simulink model "untitled"  (R2019b)
settings: Solver=VariableStepAuto  StartTime=0.0  StopTime=300  FixedStep=0.01  RelTol=1e-3
undefined symbols (not defined in the file): alpha1, alpha2, beta1, beta2, CaCO2_IC, CaO2_IC, Cbp, Cbv, Cep, Cev, Chp, Chv, Cla, Cmp, Cmv, Cpa, Cpp, Cps, Cpv, Cra, Csa, CsatCO2, CsatO2, Csp, Csv, CvCO2_IC, CvO2_IC, D1, D2, Dc, Dp, dt, Emaxlv, Emaxrv, f, fac_max, fac_min, facn, FICO2, FIO2, GcA, Gcf, GpA, Gpf, h1, h2, HR, K1, K1_tv, K2, K2_tv, kac, kElv, kErv, KH, KR, kRlv, kRrv, ksys, Kxp ... (+70)
libraries: fl_lib x42, nesl_utility x9, powerlib_meascontrol x1
(part 1 of 2)
settings Model: Creator=muratcangncr  LastModifiedBy=muratcangncr

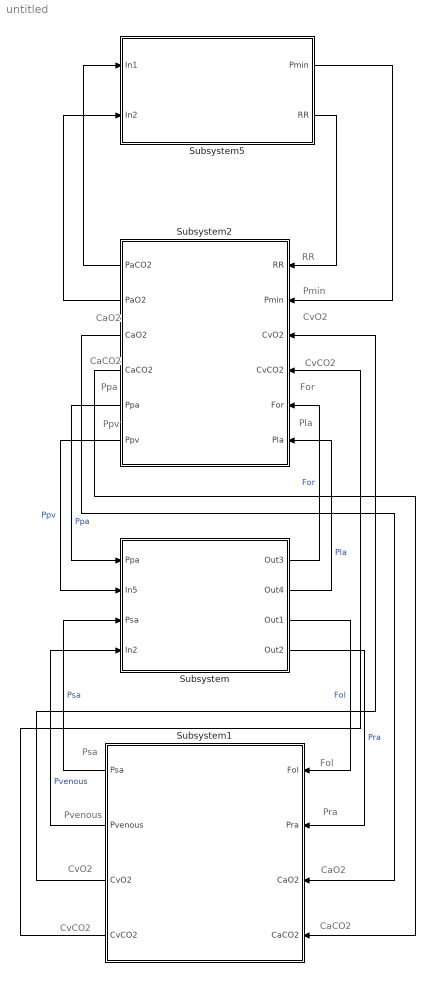
== system untitled ==
  note: Pmin
  note: RR
  note: Pvenous
  note: Psa
  note: Fol
  note: Pra
  note: CaO2
  note: CaCO2
  note: Ppa
  note: Ppv
  note: CvO2
  note: CvCO2
  note: For
  note: Pla
  note: CaO2
  note: CaCO2
  note: CvO2
  note: CvCO2
  Subsystem : Subsystem
      mask Display: image('C:\Users\muratcangncr\Desktop\MIT-Biorobotic-Heart-A1.jpg'); % Use "Edit Image" on toolstrip to change.
  Subsystem1 : Subsystem
      mask Display: image('C:\Users\muratcangncr\Desktop\systemic.jpg'); % Use "Edit Image" on toolstrip to change.
  Subsystem2 : Subsystem
      mask Display: image('C:\Users\muratcangncr\Desktop\pulmo.png'); % Use "Edit Image" on toolstrip to change.
  Subsystem5 : Subsystem
  wires:
  Subsystem/3(Out1) -> Subsystem1/1(Fol)  "Fol"
  Subsystem/4(Out2) -> Subsystem1/2(Pra)  "Pra"
  Subsystem1/1(Psa) -> Subsystem/3(Psa)  "Psa"
  Subsystem1/2(Pvenous) -> Subsystem/4(In2)  "Pvenous"
  Subsystem1/3(CvO2) -> Subsystem2/3(CvO2)
  Subsystem1/4(CvCO2) -> Subsystem2/4(CvCO2)
  Subsystem/1(Out3) -> Subsystem2/5(For)  "For"
  Subsystem/2(Out4) -> Subsystem2/6(Pla)  "Pla"
  Subsystem2/3(CaO2) -> Subsystem1/3(CaO2)
  Subsystem2/4(CaCO2) -> Subsystem1/4(CaCO2)
  Subsystem2/5(Ppa) -> Subsystem/1(Ppa)  "Ppa"
  Subsystem2/6(Ppv) -> Subsystem/2(In5)  "Ppv"
  Subsystem2/1(PaCO2) -> Subsystem5/1(In1)
  Subsystem2/2(PaO2) -> Subsystem5/2(In2)
  Subsystem5/1(Pmin) -> Subsystem2/2(Pmin)
  Subsystem5/2(RR) -> Subsystem2/1(RR)

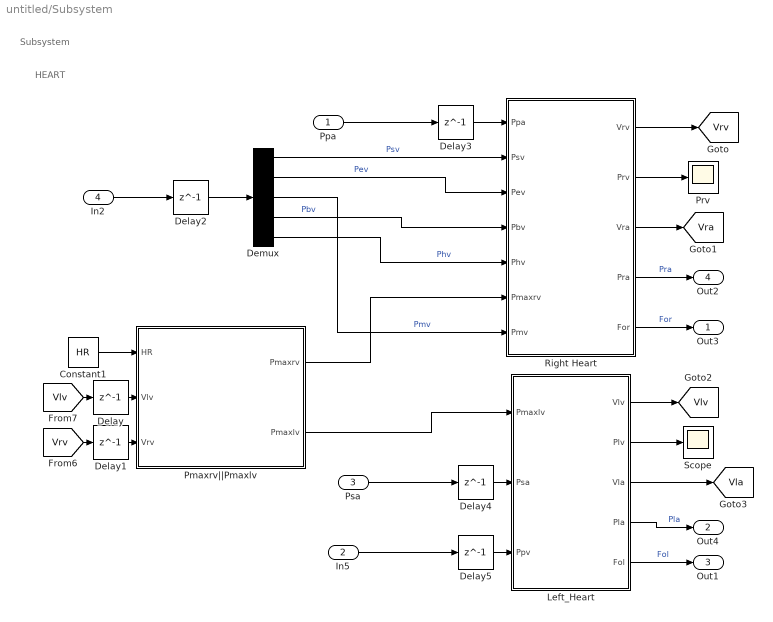
== system untitled/Subsystem ==
  note: Subsystem
  note: HEART
  Ppa : Inport
  In5 : Inport  Port=2
  Psa : Inport  Port=3
  In2 : Inport  Port=4
  Constant1 : Constant  Value=HR
  Delay{,1..5} (6 alike) : Delay  DelayLength=1  SampleTime=Tsamp
  Demux : Demux  Outputs=5
  "Left_Heart " : MATLAB Function  TreatAsAtomicUnit=on  SystemSampleTime=Tsamp
  Pmaxrv||Pmaxlv : MATLAB Function  TreatAsAtomicUnit=on  SystemSampleTime=Tsamp
  Prv : Scope
  Right Heart : MATLAB Function  TreatAsAtomicUnit=on  SystemSampleTime=Tsamp
  Scope : Scope
  Out3 : Outport
  Out4 : Outport  Port=2
  Out1 : Outport  Port=3
  Out2 : Outport  Port=4
  tag scope: Vla=global, Vlv=global, Vra=global, Vrv=global
  wires:
  Right Heart/3(Vra) -> [Vra]
  "Left_Heart "/3(Vla) -> [Vla]
  "Left_Heart "/2(Plv) -> Scope/1
  Demux/1 -> Right Heart/2(Psv)  "Psv"
  Demux/2 -> Right Heart/3(Pev)  "Pev"
  "Left_Heart "/1(Vlv) -> [Vlv]
  Right Heart/2(Prv) -> Prv/1
  Delay4/1 -> "Left_Heart "/2(Psa)
  Pmaxrv||Pmaxlv/2(Pmaxlv) -> "Left_Heart "/1(Pmaxlv)
  Constant1/1 -> Pmaxrv||Pmaxlv/1(HR)
  Pmaxrv||Pmaxlv/1(Pmaxrv) -> Right Heart/6(Pmaxrv)
  [Vlv] -> Delay/1
  Right Heart/5(For) -> Out3/1  "For"
  Right Heart/1(Vrv) -> [Vrv]
  Delay1/1 -> Pmaxrv||Pmaxlv/3(Vrv)
  Demux/5 -> Right Heart/5(Phv)  "Phv"
  [Vrv] -> Delay1/1
  Demux/3 -> Right Heart/7(Pmv)  "Pmv"
  Delay/1 -> Pmaxrv||Pmaxlv/2(Vlv)
  Demux/4 -> Right Heart/4(Pbv)  "Pbv"
  Delay5/1 -> "Left_Heart "/3(Ppv)
  Delay3/1 -> Right Heart/1(Ppa)
  Delay2/1 -> Demux/1
  In5/1 -> Delay5/1
  "Left_Heart "/4(Pla) -> Out4/1  "Pla"
  In2/1 -> Delay2/1
  Right Heart/4(Pra) -> Out2/1  "Pra"
  "Left_Heart "/5(Fol) -> Out1/1  "Fol"
  Ppa/1 -> Delay3/1
  Psa/1 -> Delay4/1

== system untitled/Subsystem1 ==
  Fol : Inport
  Pra : Inport  Port=2
  CaO2 : Inport  Port=3
  CaCO2 : Inport  Port=4
  Constant : Constant  Value=Vt0  VectorParams1D=off  SampleTime=Tsamp
  Display : Display
  Mean : powerlib_meascontrol/Measurements/Mean  Freq=1.2  Vinit=0  Ts=0
      settings: SourceProductName=Simscape Electrical
  Mux : Mux  Inputs=5
  Systemic Circ. : MATLAB Function  TreatAsAtomicUnit=on  SystemSampleTime=Tsamp
  Tissue Gas Exchange1 : Subsystem
  Psa : Outport
  Pvenous : Outport  Port=2
  CvO2 : Outport  Port=3
  CvCO2 : Outport  Port=4
  wires:
  Systemic Circ./6(Pbv) -> Mux/4
  [Vrv] -> Systemic Circ./3(Vrv)
  [Vpp] -> Systemic Circ./5(Vpp)
  Systemic Circ./5(Pmv) -> Mux/3
  [Vlv] -> Systemic Circ./8(Vlv)
  [Vla] -> Systemic Circ./10(Vla)
  Systemic Circ./4(Pev) -> Mux/2
  Systemic Circ./7(Phv) -> Mux/5
  [Vpv] -> Systemic Circ./7(Vpv)
  Systemic Circ./3(Psv) -> Mux/1  "Psv"
  [Vps] -> Systemic Circ./6(Vps)
  [Vpa] -> Systemic Circ./4(Vpa)
  Fol/1 -> Systemic Circ./1(Fol)
  Systemic Circ./1(Fsa) -> Tissue Gas Exchange1/3(Fs), Mean/1
  Constant/1 -> Systemic Circ./9(Vtotal)
  Mean/1 -> Display/1
  Pra/1 -> Systemic Circ./2(Pra)
  Tissue Gas Exchange1/2(CvCO2) -> CvCO2/1  "CvCO2"
  [Vra] -> Systemic Circ./11(Vra)
  CaCO2/1 -> Tissue Gas Exchange1/1(CaCO2)  "CaCO2"
  Systemic Circ./2(Psa) -> Psa/1  "Psa"
  Mux/1 -> Pvenous/1  "Pvenous"
  CaO2/1 -> Tissue Gas Exchange1/2(CaO2)  "CaO2"
  Tissue Gas Exchange1/1(CvO2) -> CvO2/1  "CvO2"

== system untitled/Subsystem2 ==
  RR : Inport
  Pmin : Inport  Port=2
  CvO2 : Inport  Port=3
  CvCO2 : Inport  Port=4
  For : Inport  Port=5
  Pla : Inport  Port=6
  Pulmonary : MATLAB Function  TreatAsAtomicUnit=on  SystemSampleTime=Tsamp
  Scope : Scope
  The lungs : Subsystem
  PaCO2 : Outport
  PaO2 : Outport  Port=2
  CaO2 : Outport  Port=3
  CaCO2 : Outport  Port=4
  Ppa : Outport  Port=5
  Ppv : Outport  Port=6
  tag scope: Vpa=global, Vpp=global, Vps=global, Vpv=global
  wires:
  Pulmonary/4(Vpv) -> [Vpv]
  Pulmonary/9(Fps) -> The lungs/2(Fps)
  For/1 -> Pulmonary/1(For)
  Pmin/1 -> The lungs/6(Pmin)
  CvCO2/1 -> The lungs/4(CvCO2)
  Pulmonary/5(Ppa) -> Ppa/1  "Ppa"
  Pla/1 -> Pulmonary/2(Pla)
  Pulmonary/3(Vps) -> [Vps]
  Pulmonary/1(Vpa) -> [Vpa]
  Pulmonary/2(Vpp) -> [Vpp]
  The lungs/2(PaCO2) -> PaCO2/1
  Pulmonary/7(Fpa) -> Scope/1
  Pulmonary/8(Fpp) -> The lungs/1(Fpp)
  RR/1 -> The lungs/5(RR)
  The lungs/1(PaO2) -> PaO2/1
  Pulmonary/6(Ppv) -> Ppv/1  "Ppv"
  The lungs/3(CaCO2) -> CaCO2/1
  The lungs/4(CaO2) -> CaO2/1
  CvO2/1 -> The lungs/3(CvO2)

== system untitled/Subsystem5 ==
  In1 : Inport
  In2 : Inport  Port=2
  Add1 : Sum  Inputs=+++
  Add5 : Sum  Inputs=+--
  Constant : Constant  Value=Pmin0
  Constant1 : Constant  Value=RR0
  MATLAB Function : MATLAB Function  TreatAsAtomicUnit=on
  Subsystem3 : Subsystem
  Subsystem4 : Subsystem
  Pmin : Outport
  RR : Outport  Port=2
  wires:
  Subsystem3/1(dRRp) -> Add1/3
  Add1/1 -> RR/1
  In1/1 -> Subsystem4/1(In1), MATLAB Function/1(PaCO2)
  In2/1 -> MATLAB Function/2(PaO2)
  MATLAB Function/1(fac) -> Subsystem3/1(In1)
  Subsystem4/1(dRRc) -> Add1/2
  Add5/1 -> Pmin/1
  Constant1/1 -> Add1/1
  Subsystem3/2(dPminP) -> Add5/3
  Subsystem4/2(dPminc) -> Add5/2
  Constant/1 -> Add5/1

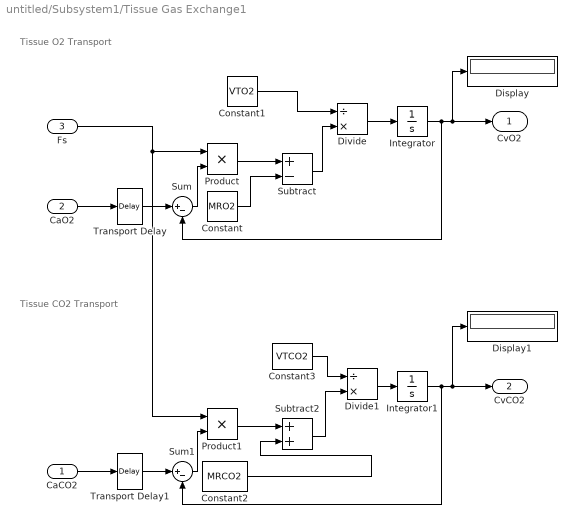
== system untitled/Subsystem1/Tissue Gas Exchange1 ==
  note: Tissue O2 Transport
  note: Tissue CO2 Transport
  CaCO2 : Inport
  CaO2 : Inport  Port=2
  Fs : Inport  Port=3
  Constant : Constant  Value=MRO2
  Constant1 : Constant  Value=VTO2
  Constant2 : Constant  Value=MRCO2
  Constant3 : Constant  Value=VTCO2
  Display : Display
  Display1 : Display
  Divide : Product  Inputs=/*
  Divide1 : Product  Inputs=/*
  Integrator : Integrator  InitialCondition=CvO2_IC
  Integrator1 : Integrator  InitialCondition=CvCO2_IC
  Product : Product
  Product1 : Product
  Subtract : Sum  Inputs=+-
  Subtract2 : Sum
  Sum : Sum  Inputs=|+-
  Sum1 : Sum  Inputs=|+-
  Transport Delay : TransportDelay  DelayTime=Tau_LT  InitialOutput=CaO2_IC
  Transport Delay1 : TransportDelay  DelayTime=Tau_LT  InitialOutput=CaCO2_IC
  CvO2 : Outport  VectorParamsAs1DForOutWhenUnconnected=off
  CvCO2 : Outport  Port=2  VectorParamsAs1DForOutWhenUnconnected=off
  wires:
  CaO2/1 -> Transport Delay/1
  Transport Delay/1 -> Sum/1
  Sum/1 -> Product/2
  Product/1 -> Subtract/1
  Divide/1 -> Integrator/1
  Integrator/1 -> Sum/2, Display/1, CvO2/1
  Subtract/1 -> Divide/2
  Constant1/1 -> Divide/1
  Product1/1 -> Subtract2/1
  Transport Delay1/1 -> Sum1/1
  Sum1/1 -> Product1/2
  Fs/1 -> Product1/1, Product/1
  Constant3/1 -> Divide1/1
  Integrator1/1 -> Sum1/2, CvCO2/1, Display1/1
  Subtract2/1 -> Divide1/2
  Divide1/1 -> Integrator1/1
  CaCO2/1 -> Transport Delay1/1
  Constant/1 -> Subtract/2
  Constant2/1 -> Subtract2/2

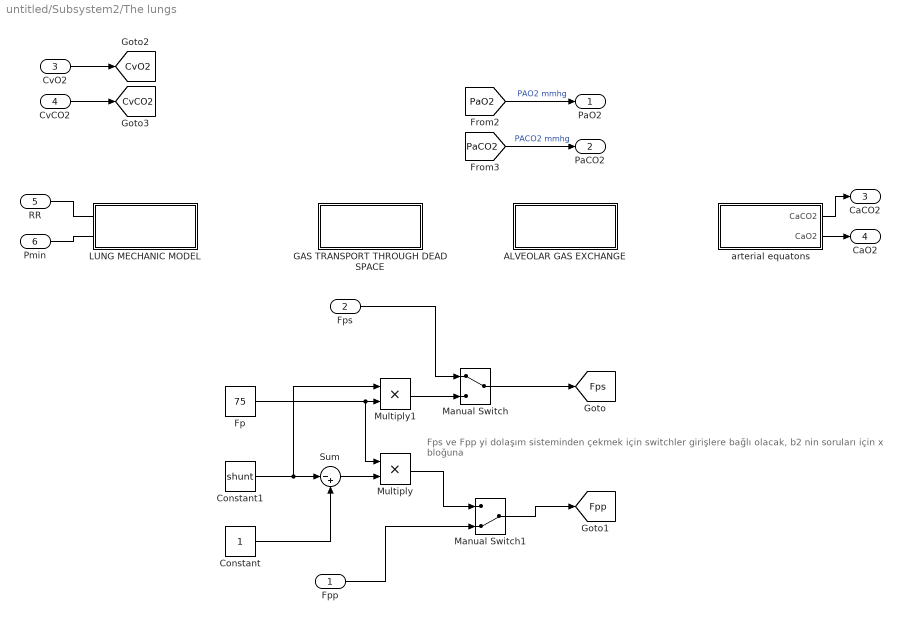
== system untitled/Subsystem2/The lungs ==
  note: Fps ve Fpp yi dolaşım sisteminden çekmek için switchler girişlere bağlı olacak, b2 nin soruları için x bloğuna
  Fpp : Inport
  Fps : Inport  Port=2
  CvO2 : Inport  Port=3
  CvCO2 : Inport  Port=4
  RR : Inport  Port=5
  Pmin : Inport  Port=6
  ALVEOLAR GAS EXCHANGE : Subsystem
  Constant : Constant
  Constant1 : Constant  Value=shunt
  Fp : Constant  Value=75
  GAS TRANSPORT THROUGH DEAD SPACE : Subsystem
  LUNG MECHANIC MODEL : Subsystem
  Manual Switch : ManualSwitch
  Manual Switch1 : ManualSwitch  CurrentSetting=0
  Multiply : Product
  Multiply1 : Product
  Sum : Sum  Inputs=|-+
  arterial equatons : Subsystem
  PaO2 : Outport  VectorParamsAs1DForOutWhenUnconnected=off
  PaCO2 : Outport  Port=2  VectorParamsAs1DForOutWhenUnconnected=off
  CaCO2 : Outport  Port=3
  CaO2 : Outport  Port=4
  tag scope: CvCO2=global, CvO2=global, Fpp=global, Fps=global
  wires:
  Pmin/1 -> ?
  RR/1 -> ?
  CvO2/1 -> [CvO2]
  CvCO2/1 -> [CvCO2]
  Constant/1 -> Sum/2
  Fpp/1 -> Manual Switch1/2
  Constant1/1 -> Multiply1/1, Sum/1
  Sum/1 -> Multiply/2
  Fp/1 -> Multiply/1, Multiply1/2
  Manual Switch1/1 -> [Fpp]
  Multiply1/1 -> Manual Switch/2
  Manual Switch/1 -> [Fps]
  Fps/1 -> Manual Switch/1
  Multiply/1 -> Manual Switch1/1
  [PaCO2] -> PaCO2/1  "PACO2 mmhg"
  [PaO2] -> PaO2/1  "PAO2 mmhg"
  arterial equatons/1(CaCO2) -> CaCO2/1
  arterial equatons/2(CaO2) -> CaO2/1

== system untitled/Subsystem5/Subsystem3 ==
  In1 : Inport
  Add2 : Sum  Inputs=+-
  Add3 : Sum  Inputs=+-
  Add4 : Sum  Inputs=+-
  Constant5 : Constant  Value=facn
  Constant6 : Constant  Value=GpA
  Constant7 : Constant  Value=TaupA
  Constant8 : Constant  Value=Gpf
  Constant9 : Constant  Value=Taupf
  Divide2 : Product  Inputs=*/
  Divide3 : Product  Inputs=*/
  Integrator2 : Integrator
  Integrator3 : Integrator
  Product2 : Product
  Product4 : Product
  Transport Delay1 : TransportDelay  DelayTime=Dp
  dRRp : Outport
  dPminP : Outport  Port=2
  wires:
  Add4/1 -> Divide3/1
  Constant7/1 -> Divide2/2
  Constant9/1 -> Divide3/2
  Product4/1 -> Add4/1
  Product2/1 -> Add3/1
  Integrator3/1 -> dRRp/1, Add4/2  "dRRp"
  Integrator2/1 -> dPminP/1, Add3/2  "dPminP"
  Add2/1 -> Product4/2, Product2/1
  Transport Delay1/1 -> Add2/1
  Constant8/1 -> Product4/1
  Divide2/1 -> Integrator2/1
  Add3/1 -> Divide2/1
  Divide3/1 -> Integrator3/1
  In1/1 -> Transport Delay1/1
  Constant5/1 -> Add2/2
  Constant6/1 -> Product2/2

== system untitled/Subsystem5/Subsystem4 ==
  In1 : Inport
  Add1 : Sum  Inputs=+-
  Add5 : Sum  Inputs=+-
  Constant : Constant  Value=PaCO2n
  Constant1 : Constant  Value=GcA
  Constant2 : Constant  Value=TaucA
  Constant3 : Constant  Value=Gcf
  Constant4 : Constant  Value=Taucf
  Divide : Product  Inputs=*/
  Divide1 : Product  Inputs=*/
  Integrator : Integrator
  Integrator1 : Integrator
  Product1 : Product
  Product3 : Product
  Sum : Sum  Inputs=-+|
  Transport Delay : TransportDelay  DelayTime=Dc
  dRRc : Outport
  dPminc : Outport  Port=2
  wires:
  Divide/1 -> Integrator/1
  Constant3/1 -> Product1/2
  Integrator1/1 -> dRRc/1, Add1/2  "dRRc"
  Add5/1 -> Divide/1
  Add1/1 -> Divide1/1
  Integrator/1 -> dPminc/1, Add5/2  "dPminc"
  Sum/1 -> Product1/1, Product3/1  "Uc"
  Constant1/1 -> Product3/2
  Product3/1 -> Add5/1
  Constant/1 -> Sum/1
  Constant2/1 -> Divide/2
  Divide1/1 -> Integrator1/1
  Constant4/1 -> Divide1/2
  Product1/1 -> Add1/1
  Transport Delay/1 -> Sum/2
  In1/1 -> Transport Delay/1

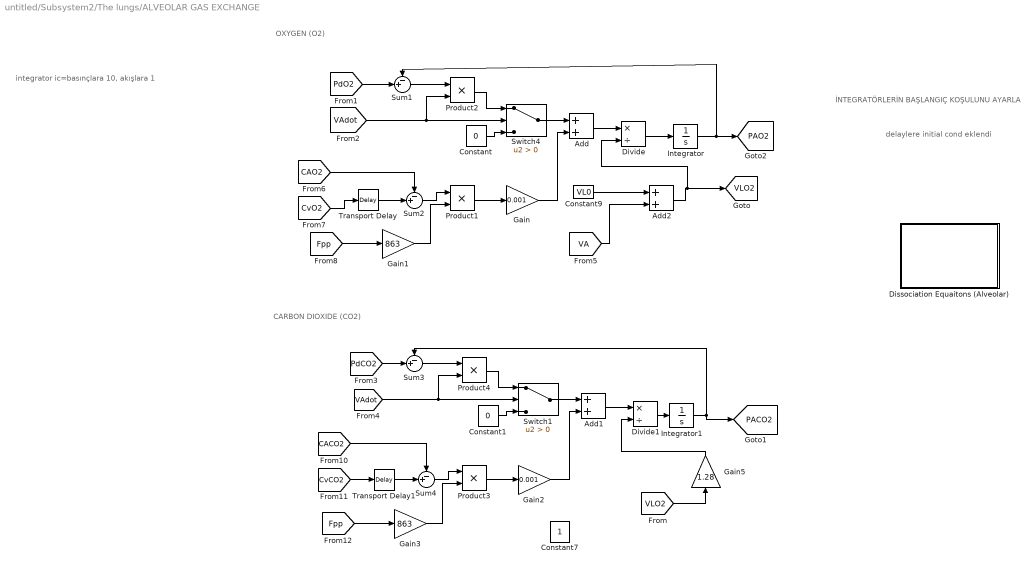
== system untitled/Subsystem2/The lungs/ALVEOLAR GAS EXCHANGE ==
  note: integrator ic=basınçlara 10, akışlara 1
  note: delaylere initial cond eklendi
  note: İNTEGRATÖRLERİN BAŞLANGIÇ KOŞULUNU AYARLA
  note: CARBON DIOXIDE (CO2)
  note: OXYGEN (O2)
  Add : Sum
  Add1 : Sum
  Add2 : Sum
  Constant : Constant  Value=0
  Constant1 : Constant  Value=0
  Constant7 : Constant
  Constant9 : Constant  Value=VL0
  Dissociation Equaitons (Alveolar) : Subsystem
  Divide : Product  Inputs=*/
  Divide1 : Product  Inputs=*/
  Gain : Gain  Gain=0.001
  Gain1 : Gain  Gain=863
  Gain2 : Gain  Gain=0.001
  Gain3 : Gain  Gain=863
  Gain5 : Gain  Gain=1.28
  Integrator : Integrator  InitialCondition=10
  Integrator1 : Integrator  InitialCondition=10
  Product{1..4} (4 alike) : Product
  Sum{1..4} (4 alike) : Sum  Inputs=-+|
  Switch1 : Switch  Criteria=u2 > Threshold
  Switch4 : Switch  Criteria=u2 > Threshold
  Transport Delay : TransportDelay  DelayTime=Tau_TL  InitialOutput=CvO2_IC
  Transport Delay1 : TransportDelay  DelayTime=Tau_TL  InitialOutput=CvCO2_IC
  tag scope: PACO2=global, PAO2=global, VLO2=global
  wires:
  [VAdot] -> Switch4/2, Product2/2
  Divide/1 -> Integrator/1
  [PdO2] -> Sum1/2
  Sum1/1 -> Product2/1
  Product2/1 -> Switch4/1
  Integrator/1 -> [PAO2], Sum1/1
  Constant/1 -> Switch4/3
  Switch4/1 -> Add/1
  Add/1 -> Divide/1
  Product1/1 -> Gain/1
  Gain/1 -> Add/2
  Sum2/1 -> Product1/1
  Gain1/1 -> Product1/2
  [CAO2] -> Sum2/1
  [CvO2] -> Transport Delay/1
  [Fpp] -> Gain1/1
  Transport Delay/1 -> Sum2/2
  Divide1/1 -> Integrator1/1
  Constant1/1 -> Switch1/3
  [VAdot] -> Switch1/2, Product4/2
  Product3/1 -> Gain2/1
  Sum3/1 -> Product4/1
  [PdCO2] -> Sum3/2
  Product4/1 -> Switch1/1
  Integrator1/1 -> [PACO2], Sum3/1
  Transport Delay1/1 -> Sum4/2
  [CACO2] -> Sum4/1
  Switch1/1 -> Add1/1
  Sum4/1 -> Product3/1
  [Fpp] -> Gain3/1
  [CvCO2] -> Transport Delay1/1
  Gain2/1 -> Add1/2
  Gain3/1 -> Product3/2
  Add1/1 -> Divide1/1
  [VA] -> Add2/2
  Constant9/1 -> Add2/1
  Add2/1 -> Divide/2, [VLO2]
  Gain5/1 -> Divide1/2
  [VLO2] -> Gain5/1

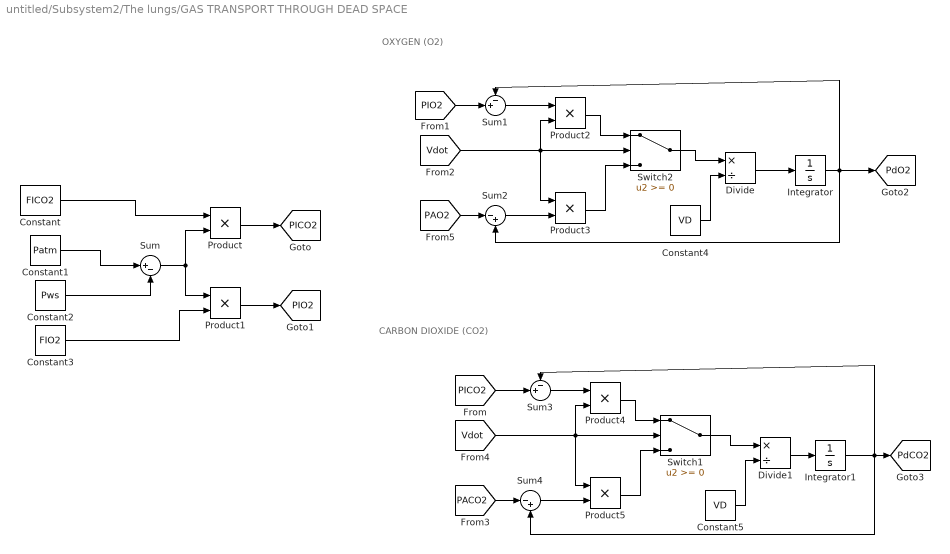
== system untitled/Subsystem2/The lungs/GAS TRANSPORT THROUGH DEAD SPACE ==
  note: CARBON DIOXIDE (CO2)
  note: OXYGEN (O2)
  Constant : Constant  Value=FICO2
  Constant1 : Constant  Value=Patm
  Constant2 : Constant  Value=Pws
  Constant3 : Constant  Value=FIO2
  Constant4 : Constant  Value=VD
  Constant5 : Constant  Value=VD
  Divide : Product  Inputs=*/
  Divide1 : Product  Inputs=*/
  Integrator : Integrator  InitialCondition=PdO2_IC
  Integrator1 : Integrator  InitialCondition=PdCO2_IC
  Product{,1..5} (6 alike) : Product
  Sum : Sum  Inputs=|+-
  Sum1 : Sum  Inputs=-+|
  Sum2 : Sum  Inputs=|-+
  Sum3 : Sum  Inputs=-+|
  Sum4 : Sum  Inputs=|-+
  Switch1 : Switch
  Switch2 : Switch
  tag scope: PICO2=global, PIO2=global, PdCO2=global, PdO2=global
  wires:
  Constant1/1 -> Sum/1
  Constant2/1 -> Sum/2
  Constant/1 -> Product/1
  Constant3/1 -> Product1/2
  Sum/1 -> Product1/1, Product/2
  Product/1 -> [PICO2]
  Product1/1 -> [PIO2]
  [PIO2] -> Sum1/2
  Sum1/1 -> Product2/1
  Product2/1 -> Switch2/1
  Switch2/1 -> Divide/1
  Constant4/1 -> Divide/2
  Divide/1 -> Integrator/1
  Integrator/1 -> Sum2/2, [PdO2], Sum1/1
  Sum2/1 -> Product3/2
  [Vdot] -> Switch2/2, Product3/1, Product2/2
  Product3/1 -> Switch2/3
  Product5/1 -> Switch1/3
  Divide1/1 -> Integrator1/1
  [PICO2] -> Sum3/2
  Switch1/1 -> Divide1/1
  Sum4/1 -> Product5/2
  [Vdot] -> Switch1/2, Product5/1, Product4/2
  Constant5/1 -> Divide1/2
  Sum3/1 -> Product4/1
  Product4/1 -> Switch1/1
  Integrator1/1 -> Sum4/2, [PdCO2], Sum3/1
  [PACO2] -> Sum4/1
  [PAO2] -> Sum2/1

== system untitled/Subsystem2/The lungs/LUNG MECHANIC MODEL ==
  Subsystem : Subsystem
  VAdot : Subsystem
  ab : Subsystem
  c : Subsystem
  d : Subsystem

== system untitled/Subsystem2/The lungs/arterial equatons ==
  CONSTANTRATION : Subsystem
  PARTİAL PRESSURES : Subsystem
  CaCO2 : Outport
  CaO2 : Outport  Port=2
  wires:
  CONSTANTRATION/1(CaCO2) -> CaCO2/1
  CONSTANTRATION/2(CaO2) -> CaO2/1

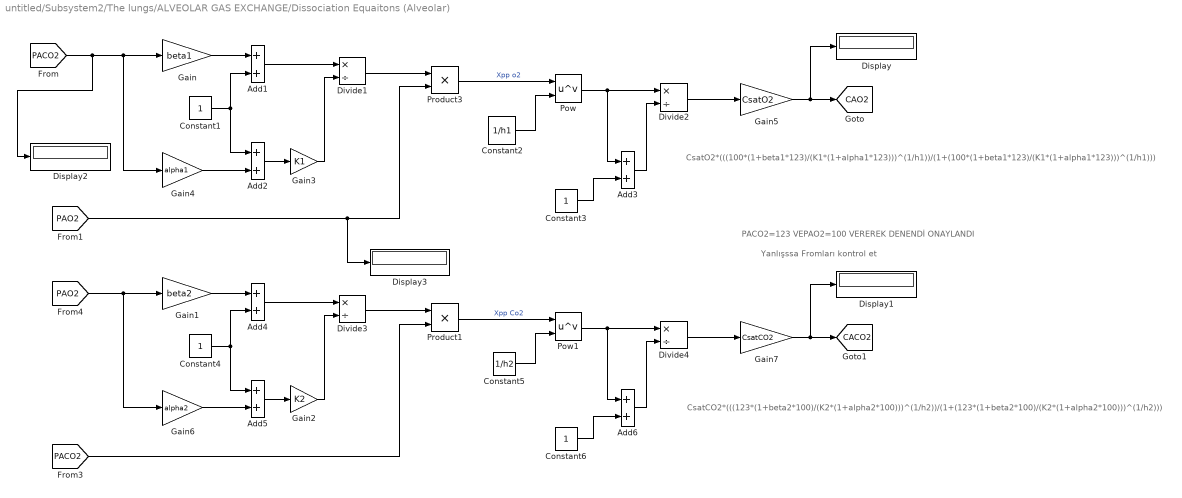
== system untitled/Subsystem2/The lungs/ALVEOLAR GAS EXCHANGE/Dissociation Equaitons (Alveolar) ==
  note: Yanlışssa Fromları kontrol et
  note: CsatO2*(((100*(1+beta1*123)/(K1*(1+alpha1*123)))^(1/h1))/(1+(100*(1+beta1*123)/(K1*(1+alpha1*123)))^(1/h1)))
  note: CsatCO2*(((123*(1+beta2*100)/(K2*(1+alpha2*100)))^(1/h2))/(1+(123*(1+beta2*100)/(K2*(1+alpha2*100)))^(1/h2)))
  note: PACO2=123 VEPAO2=100 VEREREK DENENDİ ONAYLANDI
  Add{1..6} (6 alike) : Sum
  Constant{1,3..4,6} (4 alike) : Constant
  Constant2 : Constant  Value=1/h1
  Constant5 : Constant  Value=1/h2
  Display{,1..3} (4 alike) : Display
  Divide{1..4} (4 alike) : Product  Inputs=*/
  Gain : Gain  Gain=beta1
  Gain1 : Gain  Gain=beta2
  Gain2 : Gain  Gain=K2
  Gain3 : Gain  Gain=K1
  Gain4 : Gain  Gain=alpha1
  Gain5 : Gain  Gain=CsatO2
  Gain6 : Gain  Gain=alpha2
  Gain7 : Gain  Gain=CsatCO2
  Pow : Math  Operator=pow  RndMeth=Zero  SaturateOnIntegerOverflow=on
  Pow1 : Math  Operator=pow  RndMeth=Zero  SaturateOnIntegerOverflow=on
  Product1 : Product
  Product3 : Product
  tag scope: CACO2=global, CAO2=global
  wires:
  [PACO2] -> Display2/1, Gain4/1, Gain/1
  Gain/1 -> Add1/1
  Constant1/1 -> Add2/1, Add1/2
  Add1/1 -> Divide1/1
  Gain3/1 -> Divide1/2
  Add2/1 -> Gain3/1
  Gain4/1 -> Add2/2
  Divide1/1 -> Product3/1
  [PAO2] -> Display3/1, Product3/2
  Product3/1 -> Pow/1  "Xpp o2"
  Constant2/1 -> Pow/2
  Pow/1 -> Add3/1, Divide2/1
  Constant3/1 -> Add3/2
  Add3/1 -> Divide2/2
  Divide2/1 -> Gain5/1
  Gain5/1 -> Display/1, [CAO2]
  Divide3/1 -> Product1/1
  [PACO2] -> Product1/2
  Add5/1 -> Gain2/1
  Gain6/1 -> Add5/2
  Constant4/1 -> Add5/1, Add4/2
  [PAO2] -> Gain6/1, Gain1/1
  Gain2/1 -> Divide3/2
  Gain1/1 -> Add4/1
  Pow1/1 -> Add6/1, Divide4/1
  Constant5/1 -> Pow1/2
  Gain7/1 -> Display1/1, [CACO2]
  Add6/1 -> Divide4/2
  Constant6/1 -> Add6/2
  Product1/1 -> Pow1/1  "Xpp Co2"
  Add4/1 -> Divide3/1
  Divide4/1 -> Gain7/1

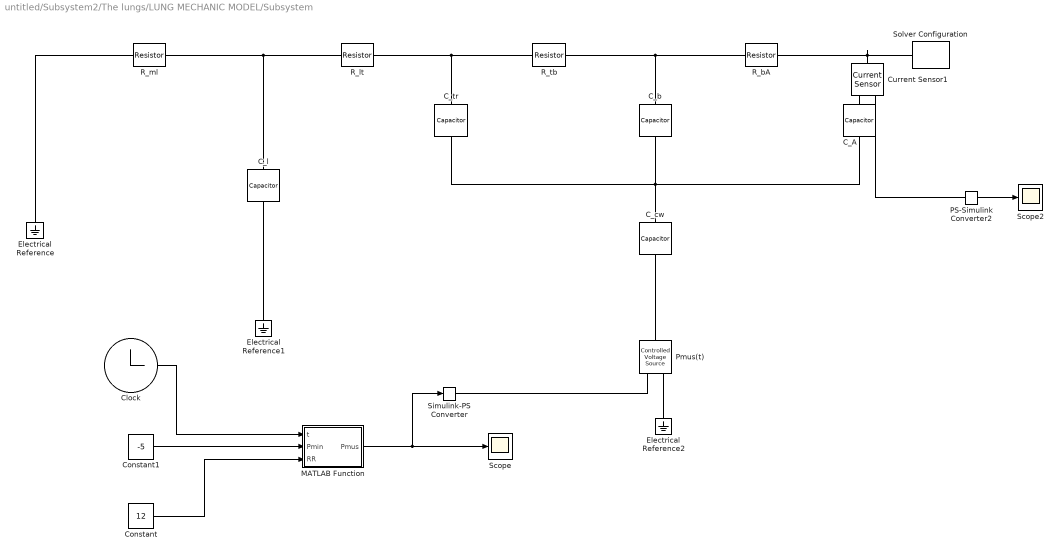
== system untitled/Subsystem2/The lungs/LUNG MECHANIC MODEL/Subsystem ==
  C_A : fl_lib/Electrical/Electrical Elements/Capacitor  c=0.175 F  r=0 Ohm  g=0 1/Ohm  i_specify=off  i_priority=None  i=0 A  i_nominal_specify=off  i_nominal_unit=A  i_nominal_value=1  v_specify=off  v_priority=None  v=0 V  v_nominal_specify=off  v_nominal_unit=V  v_nominal_value=1  vc_specify=off  vc_priority=High  vc=0 V  vc_nominal_specify=off  vc_nominal_unit=V  vc_nominal_value=1
  C_b : fl_lib/Electrical/Electrical Elements/Capacitor  c=0.0131 F  r=0 Ohm  g=0 1/Ohm  i_specify=off  i_priority=None  i=0 A  i_nominal_specify=off  i_nominal_unit=A  i_nominal_value=1  v_specify=off  v_priority=None  v=0 V  v_nominal_specify=off  v_nominal_unit=V  v_nominal_value=1  vc_specify=off  vc_priority=High  vc=0 V  vc_nominal_specify=off  vc_nominal_unit=V  vc_nominal_value=1
  C_cw : fl_lib/Electrical/Electrical Elements/Capacitor  c=0.2 F  r=0 Ohm  g=0 1/Ohm  i_specify=off  i_priority=None  i=0 A  i_nominal_specify=off  i_nominal_unit=A  i_nominal_value=1  v_specify=off  v_priority=None  v=0 V  v_nominal_specify=off  v_nominal_unit=V  v_nominal_value=1  vc_specify=off  vc_priority=High  vc=0 V  vc_nominal_specify=off  vc_nominal_unit=V  vc_nominal_value=1
  C_l : fl_lib/Electrical/Electrical Elements/Capacitor  c=0.00127 F  r=0 Ohm  g=0 1/Ohm  i_specify=off  i_priority=None  i=0 A  i_nominal_specify=off  i_nominal_unit=A  i_nominal_value=1  v_specify=off  v_priority=None  v=0 V  v_nominal_specify=off  v_nominal_unit=V  v_nominal_value=1  vc_specify=off  vc_priority=High  vc=0 V  vc_nominal_specify=off  vc_nominal_unit=V  vc_nominal_value=1
  C_tr : fl_lib/Electrical/Electrical Elements/Capacitor  c=0.00238 F  r=0 Ohm  g=0 1/Ohm  i_specify=off  i_priority=None  i=0 A  i_nominal_specify=off  i_nominal_unit=A  i_nominal_value=1  v_specify=off  v_priority=None  v=0 V  v_nominal_specify=off  v_nominal_unit=V  v_nominal_value=1  vc_specify=off  vc_priority=High  vc=0 V  vc_nominal_specify=off  vc_nominal_unit=V  vc_nominal_value=1
  Clock : Clock
      settings: Decimation=60
  Constant : Constant  Value=12
  Constant1 : Constant  Value=-5
  Current Sensor1 : fl_lib/Electrical/Electrical Sensors/Current Sensor
  Electrical Reference : fl_lib/Electrical/Electrical Elements/Electrical Reference
  Electrical Reference1 : fl_lib/Electrical/Electrical Elements/Electrical Reference
  Electrical Reference2 : fl_lib/Electrical/Electrical Elements/Electrical Reference
  MATLAB Function : MATLAB Function  TreatAsAtomicUnit=on
  PS-Simulink Converter2 : nesl_utility/PS-Simulink Converter  PhysicalDomain=network_engine_domain  SubClassName=ps_output  LeftPortType=input  RightPortType=output  PseudoPeriodic=off  Frequencies=[]  Unit=1  AffineConversion=off
  Pmus(t) : fl_lib/Electrical/Electrical Sources/Controlled Voltage Source
  R_bA : fl_lib/Electrical/Electrical Elements/Resistor  R=0.0817 Ohm  i_specify=off  i_priority=None  i=0 A  i_nominal_specify=off  i_nominal_unit=A  i_nominal_value=1  v_specify=off  v_priority=None  v=0 V  v_nominal_specify=off  v_nominal_unit=V  v_nominal_value=1
  R_lt : fl_lib/Electrical/Electrical Elements/Resistor  R=0.3369 Ohm  i_specify=off  i_priority=None  i=0 A  i_nominal_specify=off  i_nominal_unit=A  i_nominal_value=1  v_specify=off  v_priority=None  v=0 V  v_nominal_specify=off  v_nominal_unit=V  v_nominal_value=1
  R_ml : fl_lib/Electrical/Electrical Elements/Resistor  R=1.021 Ohm  i_specify=off  i_priority=None  i=0 A  i_nominal_specify=off  i_nominal_unit=A  i_nominal_value=1  v_specify=off  v_priority=None  v=0 V  v_nominal_specify=off  v_nominal_unit=V  v_nominal_value=1
  R_tb : fl_lib/Electrical/Electrical Elements/Resistor  R=0.3063 Ohm  i_specify=off  i_priority=None  i=0 A  i_nominal_specify=off  i_nominal_unit=A  i_nominal_value=1  v_specify=off  v_priority=None  v=0 V  v_nominal_specify=off  v_nominal_unit=V  v_nominal_value=1
  Scope : Scope
  Scope2 : Scope
  Simulink-PS Converter : nesl_utility/Simulink-PS Converter  PhysicalDomain=network_engine_domain  SubClassName=ps_input  LeftPortType=input  RightPortType=output  PseudoPeriodic=off  Frequencies=[]  NoiseDistribution=none  NoiseParameters=[]  Unit=1  AffineConversion=off  FilteringAndDerivatives=provide  SimscapeFilterOrder=1  InputFilterTimeConstant=0.001  UdotUserProvided=0
  Solver Configuration : nesl_utility/Solver Configuration  PhysicalDomain=network_engine_domain  SubClassName=solver  LeftPortType=input  RightPortType=generic  Tones=[]  Harmonics=[]  SimulateNoise=off  Profile=off  UseLocalSampling=off  EnableSwitchedLinearOptims=on  FrequencyDomain=off  UseCCode=off  RelTol=0.001  AbsTol=1e-06  MinStep=1e-09  ToWorkspace=off  RevertToSquareIcSolve=off  NumHomotopyIterations=100  PhasorMode=off  PhasorModeNumHarmonics=1  DoDC=off  ResidualTolerance=1e-09  UseLocalSolver=off  LocalSolverChoice=NE_BACKWARD_EULER_ADVANCER  LocalSolverSampleTime=0.001  DoFixedCost=off  MaxNonlinIter=3  MaxModeIter=2  LinearAlgebra=auto  EquationFormulation=NE_TIME_EF  DelaysMemoryBudget=1024  AutomaticFiltering=on  FilteringTimeConstant=0.001  PartitionStorageMethod=AS_NEEDED  PartitionMemoryBudget=1024  PartitionMethod=FAST
  wires:
  Constant/1 -> MATLAB Function/3(RR)
  MATLAB Function/1(Pmus) -> Scope/1, Simulink-PS Converter/1
  Constant1/1 -> MATLAB Function/2(Pmin)
  Clock/1 -> MATLAB Function/1(t)
  PS-Simulink Converter2/1 -> Scope2/1
  connections:
  R_lt/LConn1 -- R_ml/RConn1 -- C_l/LConn1
  C_A/RConn1 -- C_tr/RConn1 -- C_cw/LConn1 -- C_b/RConn1
  R_tb/LConn1 -- R_lt/RConn1 -- C_tr/LConn1
  Solver Configuration/RConn1 -- R_bA/RConn1 -- Current Sensor1/LConn1
  R_bA/LConn1 -- R_tb/RConn1 -- C_b/LConn1
  Current Sensor1/RConn1 -- PS-Simulink Converter2/LConn1
  R_ml/LConn1 -- Electrical Reference/LConn1
  Simulink-PS Converter/RConn1 -- Pmus(t)/RConn1
  Electrical Reference1/LConn1 -- C_l/RConn1
  Pmus(t)/RConn2 -- Electrical Reference2/LConn1
  Current Sensor1/RConn2 -- C_A/LConn1
  C_cw/RConn1 -- Pmus(t)/LConn1

== system untitled/Subsystem2/The lungs/LUNG MECHANIC MODEL/VAdot ==
  Clock : Clock
      settings: Decimation=5
  Constant : Constant  Value=12
  Constant1 : Constant  Value=-5
  Integrator : Integrator
  MATLAB Function : MATLAB Function  TreatAsAtomicUnit=on
  Scope : Scope  NumInputPorts=2
  Transfer Fcn : TransferFcn  Numerator=[-3.804*10^6 -2.934*10^9 -7.057*10^-5]  Denominator=[1 6996 1.213*10^7 5.615*10^9 3.273*10^10]
  tag scope: VA=global, VAdot=global
  wires:
  Clock/1 -> MATLAB Function/1(t)
  MATLAB Function/1(Pmus) -> Transfer Fcn/1  "P_mus(t)"
  Transfer Fcn/1 -> Integrator/1, [VAdot], Scope/1  "VAdot"
  Constant/1 -> MATLAB Function/3(RR)
  Constant1/1 -> MATLAB Function/2(Pmin)
  Integrator/1 -> [VA], Scope/2  "VA"

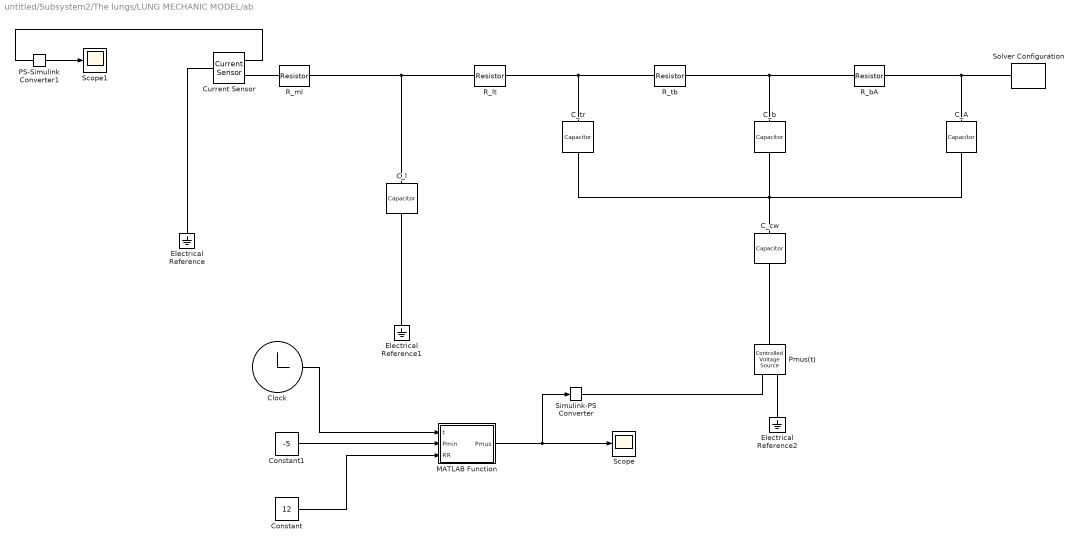
== system untitled/Subsystem2/The lungs/LUNG MECHANIC MODEL/ab ==
  C_A : fl_lib/Electrical/Electrical Elements/Capacitor  c=0.175 F  r=0 Ohm  g=0 1/Ohm  i_specify=off  i_priority=None  i=0 A  i_nominal_specify=off  i_nominal_unit=A  i_nominal_value=1  v_specify=off  v_priority=None  v=0 V  v_nominal_specify=off  v_nominal_unit=V  v_nominal_value=1  vc_specify=off  vc_priority=High  vc=0 V  vc_nominal_specify=off  vc_nominal_unit=V  vc_nominal_value=1
  C_b : fl_lib/Electrical/Electrical Elements/Capacitor  c=0.0131 F  r=0 Ohm  g=0 1/Ohm  i_specify=off  i_priority=None  i=0 A  i_nominal_specify=off  i_nominal_unit=A  i_nominal_value=1  v_specify=off  v_priority=None  v=0 V  v_nominal_specify=off  v_nominal_unit=V  v_nominal_value=1  vc_specify=off  vc_priority=High  vc=0 V  vc_nominal_specify=off  vc_nominal_unit=V  vc_nominal_value=1
  C_cw : fl_lib/Electrical/Electrical Elements/Capacitor  c=0.2 F  r=0 Ohm  g=0 1/Ohm  i_specify=off  i_priority=None  i=0 A  i_nominal_specify=off  i_nominal_unit=A  i_nominal_value=1  v_specify=off  v_priority=None  v=0 V  v_nominal_specify=off  v_nominal_unit=V  v_nominal_value=1  vc_specify=off  vc_priority=High  vc=0 V  vc_nominal_specify=off  vc_nominal_unit=V  vc_nominal_value=1
  C_l : fl_lib/Electrical/Electrical Elements/Capacitor  c=0.00127 F  r=0 Ohm  g=0 1/Ohm  i_specify=off  i_priority=None  i=0 A  i_nominal_specify=off  i_nominal_unit=A  i_nominal_value=1  v_specify=off  v_priority=None  v=0 V  v_nominal_specify=off  v_nominal_unit=V  v_nominal_value=1  vc_specify=off  vc_priority=High  vc=0 V  vc_nominal_specify=off  vc_nominal_unit=V  vc_nominal_value=1
  C_tr : fl_lib/Electrical/Electrical Elements/Capacitor  c=0.00238 F  r=0 Ohm  g=0 1/Ohm  i_specify=off  i_priority=None  i=0 A  i_nominal_specify=off  i_nominal_unit=A  i_nominal_value=1  v_specify=off  v_priority=None  v=0 V  v_nominal_specify=off  v_nominal_unit=V  v_nominal_value=1  vc_specify=off  vc_priority=High  vc=0 V  vc_nominal_specify=off  vc_nominal_unit=V  vc_nominal_value=1
  Clock : Clock
      settings: Decimation=60
  Constant : Constant  Value=12
  Constant1 : Constant  Value=-5
  Current Sensor : fl_lib/Electrical/Electrical Sensors/Current Sensor
  Electrical Reference : fl_lib/Electrical/Electrical Elements/Electrical Reference
  Electrical Reference1 : fl_lib/Electrical/Electrical Elements/Electrical Reference
  Electrical Reference2 : fl_lib/Electrical/Electrical Elements/Electrical Reference
  MATLAB Function : MATLAB Function  TreatAsAtomicUnit=on
  PS-Simulink Converter1 : nesl_utility/PS-Simulink Converter  PhysicalDomain=network_engine_domain  SubClassName=ps_output  LeftPortType=input  RightPortType=output  PseudoPeriodic=off  Frequencies=[]  Unit=1  AffineConversion=off
  Pmus(t) : fl_lib/Electrical/Electrical Sources/Controlled Voltage Source
  R_bA : fl_lib/Electrical/Electrical Elements/Resistor  R=0.0817 Ohm  i_specify=off  i_priority=None  i=0 A  i_nominal_specify=off  i_nominal_unit=A  i_nominal_value=1  v_specify=off  v_priority=None  v=0 V  v_nominal_specify=off  v_nominal_unit=V  v_nominal_value=1
  R_lt : fl_lib/Electrical/Electrical Elements/Resistor  R=0.3369 Ohm  i_specify=off  i_priority=None  i=0 A  i_nominal_specify=off  i_nominal_unit=A  i_nominal_value=1  v_specify=off  v_priority=None  v=0 V  v_nominal_specify=off  v_nominal_unit=V  v_nominal_value=1
  R_ml : fl_lib/Electrical/Electrical Elements/Resistor  R=1.021 Ohm  i_specify=off  i_priority=None  i=0 A  i_nominal_specify=off  i_nominal_unit=A  i_nominal_value=1  v_specify=off  v_priority=None  v=0 V  v_nominal_specify=off  v_nominal_unit=V  v_nominal_value=1
  R_tb : fl_lib/Electrical/Electrical Elements/Resistor  R=0.3063 Ohm  i_specify=off  i_priority=None  i=0 A  i_nominal_specify=off  i_nominal_unit=A  i_nominal_value=1  v_specify=off  v_priority=None  v=0 V  v_nominal_specify=off  v_nominal_unit=V  v_nominal_value=1
  Scope : Scope
  Scope1 : Scope
  Simulink-PS Converter : nesl_utility/Simulink-PS Converter  PhysicalDomain=network_engine_domain  SubClassName=ps_input  LeftPortType=input  RightPortType=output  PseudoPeriodic=off  Frequencies=[]  NoiseDistribution=none  NoiseParameters=[]  Unit=1  AffineConversion=off  FilteringAndDerivatives=provide  SimscapeFilterOrder=1  InputFilterTimeConstant=0.001  UdotUserProvided=0
  Solver Configuration : nesl_utility/Solver Configuration  PhysicalDomain=network_engine_domain  SubClassName=solver  LeftPortType=input  RightPortType=generic  Tones=[]  Harmonics=[]  SimulateNoise=off  Profile=off  UseLocalSampling=off  EnableSwitchedLinearOptims=on  FrequencyDomain=off  UseCCode=off  RelTol=0.001  AbsTol=1e-06  MinStep=1e-09  ToWorkspace=off  RevertToSquareIcSolve=off  NumHomotopyIterations=100  PhasorMode=off  PhasorModeNumHarmonics=1  DoDC=off  ResidualTolerance=1e-09  UseLocalSolver=off  LocalSolverChoice=NE_BACKWARD_EULER_ADVANCER  LocalSolverSampleTime=0.001  DoFixedCost=off  MaxNonlinIter=3  MaxModeIter=2  LinearAlgebra=auto  EquationFormulation=NE_TIME_EF  DelaysMemoryBudget=1024  AutomaticFiltering=on  FilteringTimeConstant=0.001  PartitionStorageMethod=AS_NEEDED  PartitionMemoryBudget=1024  PartitionMethod=FAST
  wires:
  PS-Simulink Converter1/1 -> Scope1/1
  Clock/1 -> MATLAB Function/1(t)
  Constant1/1 -> MATLAB Function/2(Pmin)
  MATLAB Function/1(Pmus) -> Scope/1, Simulink-PS Converter/1
  Constant/1 -> MATLAB Function/3(RR)
  connections:
  C_A/LConn1 -- R_bA/RConn1 -- Solver Configuration/RConn1
  R_lt/LConn1 -- R_ml/RConn1 -- C_l/LConn1
  C_A/RConn1 -- C_tr/RConn1 -- C_cw/LConn1 -- C_b/RConn1
  R_bA/LConn1 -- R_tb/RConn1 -- C_b/LConn1
  R_tb/LConn1 -- R_lt/RConn1 -- C_tr/LConn1
  Simulink-PS Converter/RConn1 -- Pmus(t)/RConn1
  R_ml/LConn1 -- Current Sensor/RConn2
  Pmus(t)/RConn2 -- Electrical Reference2/LConn1
  PS-Simulink Converter1/LConn1 -- Current Sensor/RConn1
  Current Sensor/LConn1 -- Electrical Reference/LConn1
  Electrical Reference1/LConn1 -- C_l/RConn1
  C_cw/RConn1 -- Pmus(t)/LConn1

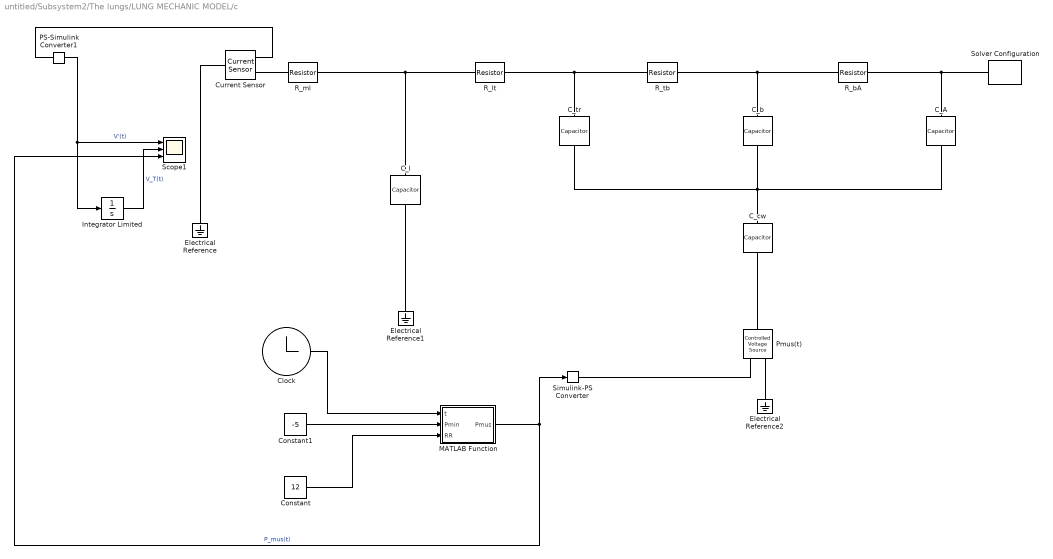
== system untitled/Subsystem2/The lungs/LUNG MECHANIC MODEL/c ==
  C_A : fl_lib/Electrical/Electrical Elements/Capacitor  c=0.175 F  r=0 Ohm  g=0 1/Ohm  i_specify=off  i_priority=None  i=0 A  i_nominal_specify=off  i_nominal_unit=A  i_nominal_value=1  v_specify=off  v_priority=None  v=0 V  v_nominal_specify=off  v_nominal_unit=V  v_nominal_value=1  vc_specify=off  vc_priority=High  vc=0 V  vc_nominal_specify=off  vc_nominal_unit=V  vc_nominal_value=1
  C_b : fl_lib/Electrical/Electrical Elements/Capacitor  c=0.0131 F  r=0 Ohm  g=0 1/Ohm  i_specify=off  i_priority=None  i=0 A  i_nominal_specify=off  i_nominal_unit=A  i_nominal_value=1  v_specify=off  v_priority=None  v=0 V  v_nominal_specify=off  v_nominal_unit=V  v_nominal_value=1  vc_specify=off  vc_priority=High  vc=0 V  vc_nominal_specify=off  vc_nominal_unit=V  vc_nominal_value=1
  C_cw : fl_lib/Electrical/Electrical Elements/Capacitor  c=0.2 F  r=0 Ohm  g=0 1/Ohm  i_specify=off  i_priority=None  i=0 A  i_nominal_specify=off  i_nominal_unit=A  i_nominal_value=1  v_specify=off  v_priority=None  v=0 V  v_nominal_specify=off  v_nominal_unit=V  v_nominal_value=1  vc_specify=off  vc_priority=High  vc=0 V  vc_nominal_specify=off  vc_nominal_unit=V  vc_nominal_value=1
  C_l : fl_lib/Electrical/Electrical Elements/Capacitor  c=0.00127 F  r=0 Ohm  g=0 1/Ohm  i_specify=off  i_priority=None  i=0 A  i_nominal_specify=off  i_nominal_unit=A  i_nominal_value=1  v_specify=off  v_priority=None  v=0 V  v_nominal_specify=off  v_nominal_unit=V  v_nominal_value=1  vc_specify=off  vc_priority=High  vc=0 V  vc_nominal_specify=off  vc_nominal_unit=V  vc_nominal_value=1
  C_tr : fl_lib/Electrical/Electrical Elements/Capacitor  c=0.00238 F  r=0 Ohm  g=0 1/Ohm  i_specify=off  i_priority=None  i=0 A  i_nominal_specify=off  i_nominal_unit=A  i_nominal_value=1  v_specify=off  v_priority=None  v=0 V  v_nominal_specify=off  v_nominal_unit=V  v_nominal_value=1  vc_specify=off  vc_priority=High  vc=0 V  vc_nominal_specify=off  vc_nominal_unit=V  vc_nominal_value=1
  Clock : Clock
      settings: Decimation=5
  Constant : Constant  Value=12
  Constant1 : Constant  Value=-5
  Current Sensor : fl_lib/Electrical/Electrical Sensors/Current Sensor
  Electrical Reference : fl_lib/Electrical/Electrical Elements/Electrical Reference
  Electrical Reference1 : fl_lib/Electrical/Electrical Elements/Electrical Reference
  Electrical Reference2 : fl_lib/Electrical/Electrical Elements/Electrical Reference
  Integrator Limited : Integrator  LimitOutput=on  UpperSaturationLimit=1  LowerSaturationLimit=0
  MATLAB Function : MATLAB Function  TreatAsAtomicUnit=on
  PS-Simulink Converter1 : nesl_utility/PS-Simulink Converter  PhysicalDomain=network_engine_domain  SubClassName=ps_output  LeftPortType=input  RightPortType=output  PseudoPeriodic=off  Frequencies=[]  Unit=1  AffineConversion=off
  Pmus(t) : fl_lib/Electrical/Electrical Sources/Controlled Voltage Source
  R_bA : fl_lib/Electrical/Electrical Elements/Resistor  R=0.0817 Ohm  i_specify=off  i_priority=None  i=0 A  i_nominal_specify=off  i_nominal_unit=A  i_nominal_value=1  v_specify=off  v_priority=None  v=0 V  v_nominal_specify=off  v_nominal_unit=V  v_nominal_value=1
  R_lt : fl_lib/Electrical/Electrical Elements/Resistor  R=0.3369 Ohm  i_specify=off  i_priority=None  i=0 A  i_nominal_specify=off  i_nominal_unit=A  i_nominal_value=1  v_specify=off  v_priority=None  v=0 V  v_nominal_specify=off  v_nominal_unit=V  v_nominal_value=1
  R_ml : fl_lib/Electrical/Electrical Elements/Resistor  R=1.021 Ohm  i_specify=off  i_priority=None  i=0 A  i_nominal_specify=off  i_nominal_unit=A  i_nominal_value=1  v_specify=off  v_priority=None  v=0 V  v_nominal_specify=off  v_nominal_unit=V  v_nominal_value=1
  R_tb : fl_lib/Electrical/Electrical Elements/Resistor  R=0.3063 Ohm  i_specify=off  i_priority=None  i=0 A  i_nominal_specify=off  i_nominal_unit=A  i_nominal_value=1  v_specify=off  v_priority=None  v=0 V  v_nominal_specify=off  v_nominal_unit=V  v_nominal_value=1
  Scope1 : Scope  NumInputPorts=3
  Simulink-PS Converter : nesl_utility/Simulink-PS Converter  PhysicalDomain=network_engine_domain  SubClassName=ps_input  LeftPortType=input  RightPortType=output  PseudoPeriodic=off  Frequencies=[]  NoiseDistribution=none  NoiseParameters=[]  Unit=1  AffineConversion=off  FilteringAndDerivatives=provide  SimscapeFilterOrder=1  InputFilterTimeConstant=0.001  UdotUserProvided=0
  Solver Configuration : nesl_utility/Solver Configuration  PhysicalDomain=network_engine_domain  SubClassName=solver  LeftPortType=input  RightPortType=generic  Tones=[]  Harmonics=[]  SimulateNoise=off  Profile=off  UseLocalSampling=off  EnableSwitchedLinearOptims=on  FrequencyDomain=off  UseCCode=off  RelTol=0.001  AbsTol=1e-06  MinStep=1e-09  ToWorkspace=off  RevertToSquareIcSolve=off  NumHomotopyIterations=100  PhasorMode=off  PhasorModeNumHarmonics=1  DoDC=off  ResidualTolerance=1e-09  UseLocalSolver=off  LocalSolverChoice=NE_BACKWARD_EULER_ADVANCER  LocalSolverSampleTime=0.001  DoFixedCost=off  MaxNonlinIter=3  MaxModeIter=2  LinearAlgebra=auto  EquationFormulation=NE_TIME_EF  DelaysMemoryBudget=1024  AutomaticFiltering=on  FilteringTimeConstant=0.001  PartitionStorageMethod=AS_NEEDED  PartitionMemoryBudget=1024  PartitionMethod=FAST
  wires:
  Constant1/1 -> MATLAB Function/2(Pmin)
  Integrator Limited/1 -> Scope1/2  "V_T(t)"
  Clock/1 -> MATLAB Function/1(t)
  PS-Simulink Converter1/1 -> Integrator Limited/1, Scope1/1  "V'(t)"
  MATLAB Function/1(Pmus) -> Simulink-PS Converter/1, Scope1/3  "P_mus(t)"
  Constant/1 -> MATLAB Function/3(RR)
  connections:
  R_lt/LConn1 -- R_ml/RConn1 -- C_l/LConn1
  R_tb/LConn1 -- R_lt/RConn1 -- C_tr/LConn1
  R_bA/LConn1 -- R_tb/RConn1 -- C_b/LConn1
  C_A/RConn1 -- C_tr/RConn1 -- C_cw/LConn1 -- C_b/RConn1
  C_A/LConn1 -- R_bA/RConn1 -- Solver Configuration/RConn1
  R_ml/LConn1 -- Current Sensor/RConn2
  Electrical Reference1/LConn1 -- C_l/RConn1
  PS-Simulink Converter1/LConn1 -- Current Sensor/RConn1
  Current Sensor/LConn1 -- Electrical Reference/LConn1
  C_cw/RConn1 -- Pmus(t)/LConn1
  Pmus(t)/RConn2 -- Electrical Reference2/LConn1
  Simulink-PS Converter/RConn1 -- Pmus(t)/RConn1

== system untitled/Subsystem2/The lungs/LUNG MECHANIC MODEL/d ==
  Clock : Clock
      settings: Decimation=5
  Constant : Constant  Value=12
  Constant1 : Constant  Value=-5
  Integrator Limited : Integrator  LimitOutput=on  UpperSaturationLimit=1  LowerSaturationLimit=0
  MATLAB Function : MATLAB Function  TreatAsAtomicUnit=on
  Scope : Scope  NumInputPorts=2
  Transfer Fcn : TransferFcn  Numerator=[-2289 -6.01*10^6 -3.193*10^9 0]  Denominator=[1 6996 1.213*10^7 5.615*10^9 3.273*10^10]
  tag scope: Vdot=global
  wires:
  MATLAB Function/1(Pmus) -> Transfer Fcn/1  "P_mus(t)"
  Constant/1 -> MATLAB Function/3(RR)
  Clock/1 -> MATLAB Function/1(t)
  Integrator Limited/1 -> Scope/2  "V_T(t)"
  Constant1/1 -> MATLAB Function/2(Pmin)
  Transfer Fcn/1 -> Integrator Limited/1, [Vdot], Scope/1  "V'(t)"

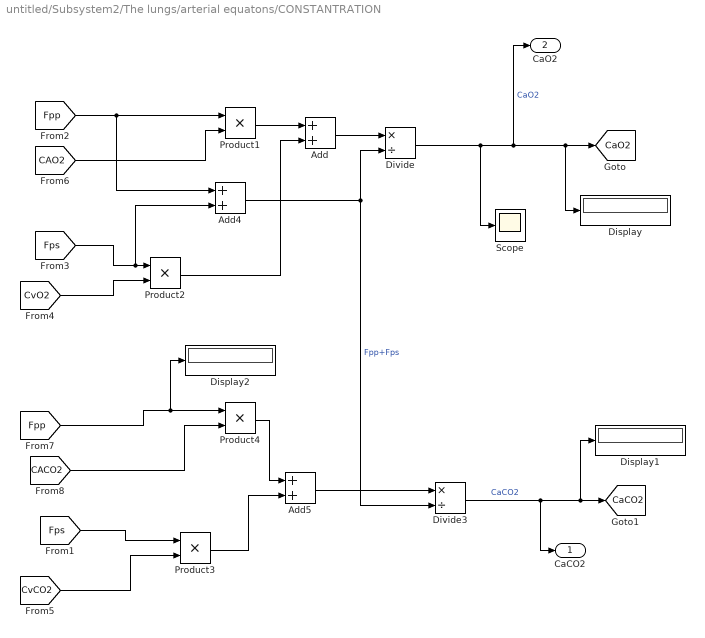
== system untitled/Subsystem2/The lungs/arterial equatons/CONSTANTRATION ==
  Add : Sum
  Add4 : Sum
  Add5 : Sum
  Display : Display
  Display1 : Display
  Display2 : Display
  Divide : Product  Inputs=*/
  Divide3 : Product  Inputs=*/
  Product{1..4} (4 alike) : Product
  Scope : Scope
  CaCO2 : Outport
  CaO2 : Outport  Port=2
  tag scope: CaCO2=global, CaO2=global
  wires:
  [Fpp] -> Product1/1, Add4/1
  [CAO2] -> Product1/2
  Product3/1 -> Add5/2
  Product4/1 -> Add5/1
  [Fps] -> Product3/1
  Add/1 -> Divide/1
  Divide3/1 -> CaCO2/1, Display1/1, [CaCO2]  "CaCO2"
  Add5/1 -> Divide3/1
  [CvO2] -> Product2/2
  [Fps] -> Add4/2, Product2/1
  [Fpp] -> Display2/1, Product4/1
  [CvCO2] -> Product3/2
  Add4/1 -> Divide3/2, Divide/2  "Fpp+Fps"
  [CACO2] -> Product4/2
  Divide/1 -> Scope/1, CaO2/1, Display/1, [CaO2]  "CaO2"
  Product1/1 -> Add/1
  Product2/1 -> Add/2

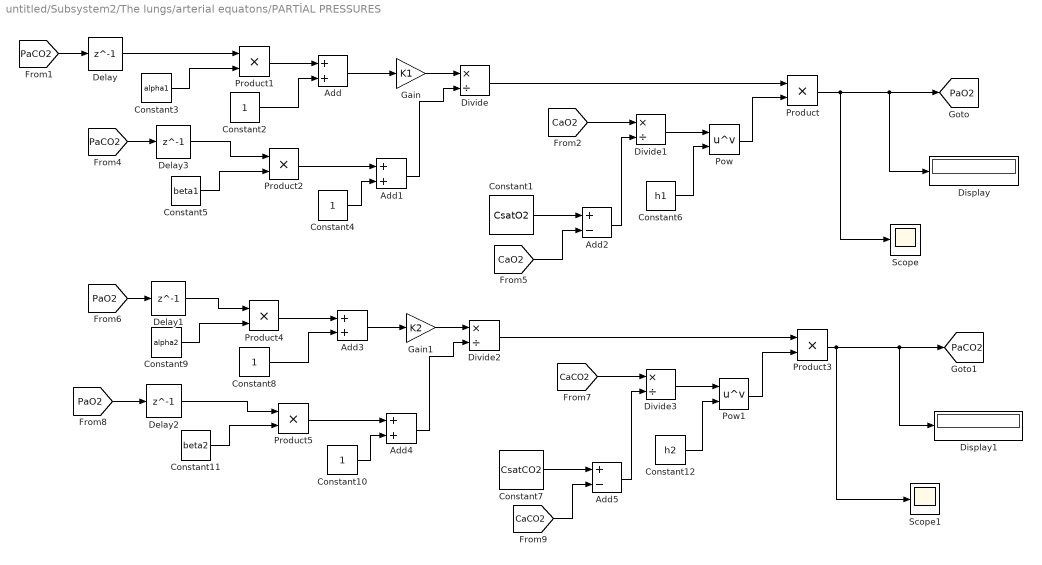
== system untitled/Subsystem2/The lungs/arterial equatons/PARTİAL PRESSURES ==
  Add{,1,3..4} (4 alike) : Sum
  Add2 : Sum  Inputs=+-
  Add5 : Sum  Inputs=+-
  Constant1 : Constant  Value=CsatO2
  Constant{2,4,8,10} (4 alike) : Constant
  Constant11 : Constant  Value=beta2
  Constant12 : Constant  Value=h2
  Constant3 : Constant  Value=alpha1
  Constant5 : Constant  Value=beta1
  Constant6 : Constant  Value=h1
  Constant7 : Constant  Value=CsatCO2
  Constant9 : Constant  Value=alpha2
  Delay{,1..3} (4 alike) : Delay  DelayLength=1  SampleTime=Tsamp
  Display : Display
  Display1 : Display
  Divide{,1..3} (4 alike) : Product  Inputs=*/
  Gain : Gain  Gain=K1
  Gain1 : Gain  Gain=K2
  Pow : Math  Operator=pow  RndMeth=Zero  SaturateOnIntegerOverflow=on
  Pow1 : Math  Operator=pow  RndMeth=Zero  SaturateOnIntegerOverflow=on
  Product{,1..5} (6 alike) : Product
  Scope : Scope
  Scope1 : Scope
  tag scope: PaCO2=global, PaO2=global
  wires:
  [PaCO2] -> Delay/1
  Constant2/1 -> Add/2
  Constant4/1 -> Add1/2
  Add1/1 -> Divide/2
  Product1/1 -> Add/1
  Constant3/1 -> Product1/2
  Add/1 -> Gain/1
  Gain/1 -> Divide/1
  [PaCO2] -> Delay3/1
  Constant5/1 -> Product2/2
  Product2/1 -> Add1/1
  [CaO2] -> Divide1/1
  Constant1/1 -> Add2/1
  [CaO2] -> Add2/2
  Add2/1 -> Divide1/2
  Divide/1 -> Product/1
  Divide1/1 -> Pow/1
  Constant6/1 -> Pow/2
  Pow/1 -> Product/2
  Product/1 -> Scope/1, Display/1, [PaO2]
  Gain1/1 -> Divide2/1
  [PaO2] -> Delay2/1
  [PaO2] -> Delay1/1
  Constant12/1 -> Pow1/2
  Constant7/1 -> Add5/1
  Product5/1 -> Add4/1
  Product3/1 -> Scope1/1, Display1/1, [PaCO2]
  Constant8/1 -> Add3/2
  Add5/1 -> Divide3/2
  Product4/1 -> Add3/1
  Add4/1 -> Divide2/2
  [CaCO2] -> Divide3/1
  Constant9/1 -> Product4/2
  Pow1/1 -> Product3/2
  Divide3/1 -> Pow1/1
  Constant11/1 -> Product5/2
  Divide2/1 -> Product3/1
  Add3/1 -> Gain1/1
  Constant10/1 -> Add4/2
  [CaCO2] -> Add5/2
  Delay/1 -> Product1/1
  Delay1/1 -> Product4/1
  Delay2/1 -> Product5/1
  Delay3/1 -> Product2/1

== matlab function untitled/Subsystem/Right Heart ==
  data: Ppa input; Vrv output; Psv input; Pev input; Pbv input; Phv input; Pmaxrv input; Pmv input; Prv output; Vra output; Pra output; For output; Rra parameter; Cra parameter; Rsv parameter; Rev parameter; Rmv parameter; Rbv parameter; Rhv parameter; kRrv parameter; dt parameter; Vura parameter; Vurv parameter
function [Vrv, Prv, Vra, Pra, For]= fcn(Ppa, Psv, Pev, Pbv, Phv, Pmaxrv, Pmv, Rra, Cra, Rsv, Rev, Rmv, Rbv, Rhv, kRrv, dt, Vura,Vurv) 
persistent Pra_1 Vrv_1;

if isempty(Pra_1)
    Pra_1 = 5.0;
    Vrv_1 = Vurv;
   
end


Rrv = max(1e-3, kRrv*Pmaxrv);


For = max(0, (Pmaxrv-Ppa)/ Rrv);


Prv = Pmaxrv-Rrv*For;


Fir = max(0, (Pra_1 - Prv) / Rra);


RHS = (((Psv - Pra_1) / Rsv) + ((Pev - Pra_1) / Rev) + ((Pmv - Pra_1) / Rmv) + ((Pbv - Pra_1) / Rbv) + ((Phv - Pra_1) / Rhv - Fir))/Cra;
Pra = Pra_1 + dt*RHS;
Vra = Pra_1*Cra + Vura;


RHS = (Fir - For);
Vrv = Vrv_1 + dt*RHS;

%Assignments
Pra_1 = Pra;
Vrv_1 = Vrv;


end

== matlab function untitled/Subsystem/Left_Heart  ==
  data: Pmaxlv input; Vlv output; Psa input; Ppv input; Plv output; Vla output; Pla output; Fol output; Rpv parameter; Cla parameter; Rla parameter; kRlv parameter; Vulv parameter; Vula parameter; dt parameter


function [Vlv, Plv, Vla, Pla, Fol] = fcn(Pmaxlv, Psa, Ppv, Rpv, Cla, Rla, kRlv, Vulv, Vula, dt)
persistent Pla_1 Vlv_1;

if isempty(Pla_1)
    Pla_1 = 10.0;
    Vlv_1 = Vulv;
end

%Eq A.1.4
Rlv = kRlv * Pmaxlv;
%Eq A.1.10
Fol = max(0, (Pmaxlv - Psa)/Rlv);
%Eq A.1.3
Plv = Pmaxlv - Rlv*Fol;
%Eq A.1.2
Fil = max(0,(Pla_1 - Plv)/Rla);
%Diff eq A.1.1
RHS = (((Ppv - Pla_1)/Rpv) - Fil)/Cla;
Pla = Pla_1 + dt*RHS;
Vla = Pla*Cla + Vula;
%Eq A.1.9
RHS = (Fil - Fol);
Vlv = Vlv_1 + dt*RHS;

%Assignments
Pla_1 = Pla;
Vlv_1 = Vlv;

end

== matlab function untitled/Subsystem/Pmaxrv||Pmaxlv ==
  data: HR input; Pmaxrv output; Vlv input; Vrv input; Pmaxlv output; Tsys0 parameter; ksys parameter; Vulv parameter; Vurv parameter; kElv parameter; kErv parameter; P0rv parameter; P0lv parameter; Emaxlv parameter; Emaxrv parameter; dt parameter
function [Pmaxrv, Pmaxlv] = fcn(HR, Vlv, Vrv, Tsys0, ksys, Vulv, Vurv, kElv, kErv, P0rv, P0lv, Emaxlv, Emaxrv, dt)
persistent ut_1;

if isempty(ut_1)
    ut_1 = 0.0;
end

%Heart period
T = 60/HR;
% A.1.8
Tsys = Tsys0 - ksys/T;

ut = ut_1 + dt*1/T;
% A.1.6
if ut_1 >= Tsys/T
    Phi = 0;
else
    Phi = sin(pi*T*ut_1 / Tsys)^2;
end
% A.1.7
if ut > 1
    ut_1 = 0.0;
else 
    ut_1 = ut;
end
%Outputs A.1.5
Pmaxrv = Phi * Emaxrv * (Vrv-Vurv) + (1-Phi) * P0rv * (exp(kErv*Vrv) -1);
Pmaxlv = Phi * Emaxlv * (Vlv-Vulv) + (1-Phi) * P0lv * (exp(kElv*Vlv) -1);
end

== matlab function untitled/Subsystem1/Systemic Circ. ==
  data: Fol input; Fsa output; Pra input; Vrv input; Vpa input; Vpp input; Vps input; Vpv input; Vlv input; Psa output; Psv output; Pev output; Pmv output; Pbv output; Phv output; Rev parameter; Rsv parameter; Rtv0 parameter; Vtvmax parameter; KR parameter; Vutv parameter; K1_tv parameter; D1 parameter; Vtvmin parameter; Cep parameter; Cmp parameter; Cbp parameter; Chp parameter; Kxp parameter; Kxv parameter; D2 parameter; K2_tv parameter; Vubp parameter; Vump parameter; Vuep parameter; Vusp parameter; Vusa parameter; Chv parameter; Cbv parameter; Cmv parameter; Csv parameter; Rhv parameter; Rbv parameter; Rmv parameter; dt parameter; Csa parameter; Rsp parameter; Rep parameter; Rmp parameter; Rbp parameter; Rhp parameter; Csp parameter; Vuev parameter; Cev parameter; Vuhv parameter; Vubv parameter; Vumv parameter; Vusv parameter; Vuhp parameter; Rsa parameter; Lsa parameter; Vtotal input; Vla input; Vra input
function [Fsa, Psa, Psv, Pev, Pmv, Pbv, Phv] = fcn(Fol, Pra, Vrv, Vpa, Vpp, Vps, Vpv, Vlv, Rev, Rsv, Rtv0, Vtvmax, KR, Vutv, K1_tv, D1, Vtvmin, Cep, Cmp, Cbp, Chp, Kxp, Kxv, D2, K2_tv, Vubp, Vump, Vuep, Vusp, Vusa, Chv, Cbv, Cmv, Csv, Rhv, Rbv, Rmv, dt, Csa, Rsp, Rep, Rmp, Rbp, Rhp, Csp, Vuev, Cev, Vuhv, Vubv, Vumv, Vusv, Vuhp, Rsa, Lsa, Vtotal,Vla,Vra)
persistent Psa_1 Psp_1 Psv_1 Pev_1 Pmv_1 Pbv_1 Phv_1 Fsa_1 Vtv_1;

if isempty(Psa_1)
    Psa_1 = 80.0;
    Psp_1 = 80.0;
    Psv_1 = 7.5;
    Pev_1 = 0.5;
    Pmv_1 = 7.5;
    Pbv_1 = 7.5;
    Phv_1 = 7.5;
    Fsa_1 = 1.0;
    Vtv_1 = Vtvmin;
end

%Diff eq A.2.2
RHS = (Psa_1 -  Psp_1 - Rsa*Fsa_1) /Lsa;
Fsa = Fsa_1 + dt*RHS;

%Diff eq A.2.1
RHS = (Fol-Fsa)/Csa;
Psa = Psa_1 + dt*RHS;

%Diff eq A.2.5
Fsp = max(0, ((Psp_1 - Psv_1) /Rsp));
Fep = max(0, ((Psp_1 - Pev_1) /Rep));
Fmp = max(0, ((Psp_1 - Pmv_1) /Rmp));
Fbp = max(0, ((Psp_1 - Pbv_1) /Rbp));
Fhp = max(0, ((Psp_1 - Phv_1) /Rhp));
%Diff Eq A.2.4
RHS = (Fsa - Fsp - Fep - Fmp - Fbp - Fhp) / (Csp + Cep + Cmp + Cbp + Chp);
Psp = Psp_1 + dt*RHS;

%Eq A.2.15
Phi = Kxp / exp((Vtv_1 / Kxv)-1);
if Vtv_1 < Vutv
    Ptv = D2 + K2_tv*exp(Vtv_1 / Vtvmin) - Phi;
else
    Ptv = D1 + K1_tv * (Vtv_1 - Vutv) - Phi;
end

%Eq Rtv A.2.12
Rtv = KR * (Vtvmax/Vtv_1)^2 + Rtv0;
%Eq A.2.13
Fsv = max(0, ((Psv_1 - Ptv) / Rsv));
Fev = max(0, ((Pev_1 - Ptv) / Rev));
Fmv = max(0, ((Pmv_1 - Ptv) / Rmv));
Fbv = max(0, ((Pbv_1 - Ptv) / Rbv));
Fhv = max(0, ((Phv_1 - Ptv) / Rhv));
% Eq Ftv A.2.12
Ftv = (Ptv - Pra) / Rtv;

% Diff Eq A.2.12
RHS = (Fsv + Fev + Fmv + Fbv + Fhv - Ftv);
Vtv = Vtv_1 + dt*RHS;

%Diff eq A.2.7
RHS = (Fsp - Fsv) / Csv;
Psv = Psv_1 + dt*RHS;
%Diff eq A.2.8
RHS = (Fmp - Fmv) / Cmv;
Pmv = Pmv_1 + dt*RHS;
%Diff eq A.2.9
RHS = (Fbp - Fbv) / Cbv;
Pbv = Pbv_1 + dt*RHS;
%Diff eq A.2.10
RHS = (Fhp - Fhv) / Chv;
Phv = Phv_1 + dt*RHS;

%Eq A.2.3
Vsa = Csa*Psa + Vusa;
%Eq A.2.6
Vsp = Csp*Psp + Vusp;
Vep = Csp*Psp + Vuep;
Vmp = Csp*Psp + Vump;
Vbp = Csp*Psp + Vubp;
Vhp = Csp*Psp + Vuhp;

%Eq A.2.14
Vsv = Csv*Psv + Vusv;
Vmv = Cmv*Pmv + Vumv;
Vbv = Cbv*Pbv + Vubv;
Vhv = Chv*Phv + Vuhv;



%Eq A.2.11
Pev = (Vtotal - Vsa - Vhp - Vbp - Vmp - Vsp - Vep - Vhv - Vbv - Vmv ...
    - Vsv - Vuev - Vtv - Vra - Vrv - Vpa - Vpp - Vps - Vpv - Vla ...
    - Vlv) / Cev;

%Assignments
Fsa_1 = Fsa;
Psa_1 = Psa;
Psp_1 = Psp;
Psv_1 = Psv;
Pmv_1 = Pmv;
Phv_1 = Phv;
Pbv_1 = Pbv;
Pev_1 = Pev;
Vtv_1 = Vtv;

end

== matlab function untitled/Subsystem2/Pulmonary ==
  data: For input; Vpa output; Pla input; Vpp output; Vps output; Vpv output; Ppa output; Ppv output; Fpa output; Fpp output; Fps output; Cpa parameter; Rpa parameter; Lpa parameter; Vupa parameter; Vupp parameter; Vups parameter; Vupv parameter; Rpp parameter; Rps parameter; Rpv parameter; dt parameter; Cpp parameter; Cps parameter; Cpv parameter
function [Vpa, Vpp, Vps, Vpv, Ppa, Ppv, Fpa, Fpp, Fps]  = fnc(For, Pla, Cpa, Rpa, Lpa, Vupa, Vupp, Vups, Vupv, Rpp, Rps, Rpv, dt, Cpp, Cps, Cpv)
persistent Ppa_1 Ppp_1 Ppv_1 Fpa_1;
if isempty(Ppa_1)
    Ppa_1 = 5.0;
    Ppp_1 = 5.0;
    Ppv_1 = 5.0;
    Fpa_1 = 0.1;
end

%Diff eq A.2.17
RHS = (Ppa_1 - Ppp_1 - Rpa*Fpa_1)/Lpa;
Fpa = Fpa_1 + dt*RHS;

%Diff eq A.2.16
RHS = (For - Fpa)/Cpa;
Ppa = Ppa_1 + dt*RHS;

%Diff eq A.2.20
Fpp = max(0.1, ((Ppp_1 - Ppv_1)/Rpp));
Fps = max(0.1, ((Ppp_1 - Ppv_1)/Rps));

%Diff eq A.2.19
RHS = (Fpa - Fps - Fpp) / (Cpp + Cps);
Ppp = Ppp_1 + dt*RHS;

%Eq A.2.23
Fpv = ((Ppv_1 - Pla) / Rpv);

%Diff eq A.2.22
RHS = (Fpp + Fps - Fpv) / Cpv;
Ppv = Ppv_1 + dt*RHS;

%Eq A.2.18
Vpa = Cpa*Ppa + Vupa;
%Eq A.2.21
Vpp = Cpp*Ppp + Vupp;
Vps = Cps*Ppp + Vups;
%Eq A.2.24
Vpv = Cpv*Ppv + Vupv;

%Assignments
Ppa_1 = Ppa;
Ppp_1 = Ppp;
Ppv_1 = Ppv;
Fpa_1 = Fpa;

end

== matlab function untitled/Subsystem2/The lungs/LUNG MECHANIC MODEL/Subsystem/MATLAB Function ==
  data: t input; Pmin input; RR input; Pmus output
function Pmus = fcn(t, Pmin, RR)
IEratio = 1/2;
T=(60/RR);
Te = T / (IEratio + 1);
Ti = IEratio * Te;
tau=Te/10;
if (rem(t,T)) < Ti
u=Pmin*(T*rem(t,T)-rem(t,T)^2)/(Ti*Te);
else
u=Pmin*(exp(-(rem(t,T)-Ti)/tau)-exp(-Te/tau))/(1-exp(-Te/tau));
end
Pmus = u;
end

== matlab function untitled/Subsystem2/The lungs/LUNG MECHANIC MODEL/VAdot/MATLAB Function ==
  data: t input; Pmin input; RR input; Pmus output
function Pmus = fcn(t, Pmin, RR)
IEratio = 1/2;
T=(60/RR);
Te = T / (IEratio + 1);
Ti = IEratio * Te;
tau=Te/10;
if (rem(t,T)) < Ti
u=Pmin*(T*rem(t,T)-rem(t,T)^2)/(Ti*Te);
else
u=Pmin*(exp(-(rem(t,T)-Ti)/tau)-exp(-Te/tau))/(1-exp(-Te/tau));
end
Pmus = u;
end

== matlab function untitled/Subsystem2/The lungs/LUNG MECHANIC MODEL/ab/MATLAB Function ==
  data: t input; Pmin input; RR input; Pmus output
function Pmus = fcn(t, Pmin, RR)
IEratio = 1/2;
T=(60/RR);
Te = T / (IEratio + 1);
Ti = IEratio * Te;
tau=Te/10;
if (rem(t,T)) < Ti
u=Pmin*(T*rem(t,T)-rem(t,T)^2)/(Ti*Te);
else
u=Pmin*(exp(-(rem(t,T)-Ti)/tau)-exp(-Te/tau))/(1-exp(-Te/tau));
end
Pmus = u;
end

== matlab function untitled/Subsystem2/The lungs/LUNG MECHANIC MODEL/c/MATLAB Function ==
  data: t input; Pmin input; RR input; Pmus output
function Pmus = fcn(t, Pmin, RR)
IEratio = 1/2;
T=(60/RR);
Te = T / (IEratio + 1);
Ti = IEratio * Te;
tau=Te/10;
if (rem(t,T)) < Ti
u=Pmin*(T*rem(t,T)-rem(t,T)^2)/(Ti*Te);
else
u=Pmin*(exp(-(rem(t,T)-Ti)/tau)-exp(-Te/tau))/(1-exp(-Te/tau));
end
Pmus = u;
end

== matlab function untitled/Subsystem2/The lungs/LUNG MECHANIC MODEL/d/MATLAB Function ==
  data: t input; Pmin input; RR input; Pmus output
function Pmus = fcn(t, Pmin, RR)
IEratio = 1/2;
T=(60/RR);
Te = T / (IEratio + 1);
Ti = IEratio * Te;
tau=Te/10;
if (rem(t,T)) < Ti
u=Pmin*(T*rem(t,T)-rem(t,T)^2)/(Ti*Te);
else
u=Pmin*(exp(-(rem(t,T)-Ti)/tau)-exp(-Te/tau))/(1-exp(-Te/tau));
end
Pmus = u;
end
